simulink model "Manipulator"  (R2021a)
settings: Solver=VariableStepAuto  StartTime=0.0  StopTime=10.0  RelTol=1e-3
model workspace: external: MATLAB File /Users/nikodemlazarz/Documents/inzynierka/matlab/rotob /simscape/robot_DataFile.m (data not in the file)
undefined symbols (not defined in the file): S, smiData, Tx, Ty, Tz, X, x0, x1, Y, y0, y1, Z, z0, z1
libraries: sm_lib x20, simulink x8, nesl_utility x4
settings Model: Creator=nikod  LastModifiedBy=nikodemlazarz
settings ExplorerConfigSet: InternalSimMechanicsExplorerSettings="<ExplorerConfiguration><canonicalview>aerospace</canonicalview><AnimationSetting><BasePlaybackSpeed>1.0</BasePlaybackSpeed><PlaybackSpeedFactor>1.0</PlaybackSpeedFactor></AnimationSetting><TilePanel><TileInfo><Tiles Columns=\"1\" Count=\"1\" Rows=\"1\"><Column Weight=\"1\"/><Row Weight=\"1\"/><Tile Height=\"1\" Width=\"1\" X=\"0\" Y=\"0\"/></Tiles></TileInfo><SceneInfo><SceneViewer><BGColor><R>0.60000002384185791</R><G>0.60000002384185791</G><B>0.60000002384185791</B></BGColor><Camera><DoPerspective>off</DoPerspective><Position><X>2.62972255265206911</X><Y>-2.13592780536878957</Y><Z>-1.22972255243143036</Z></Position><Center><X>1.29999996897715486</X><Y>-0.806205221693875429</Y><Z>0.100000031243483445</Z></Center><Up><X>-0.408248290463863073</X><Y>0.408248290463863073</Y><Z>-0.816496580927726145</Z></Up><ViewLimDist>1</ViewLimDist><YLim>2.00898007835833559</YLim><XLim>1.8936319398880006</XLim></Camera></SceneViewer></SceneInfo></TilePanel><MechEditorPanel><Cameras/><GfxPanelCameraMap/><VideoCreator><PlaybackSpeedRatio>1.0</PlaybackSpeedRatio><FrameRate>30</FrameRate><VideoFormat>Motion JPEG AVI</VideoFormat><FrameSize>auto</FrameSize></VideoCreator></MechEditorPanel></ExplorerConfiguration>"

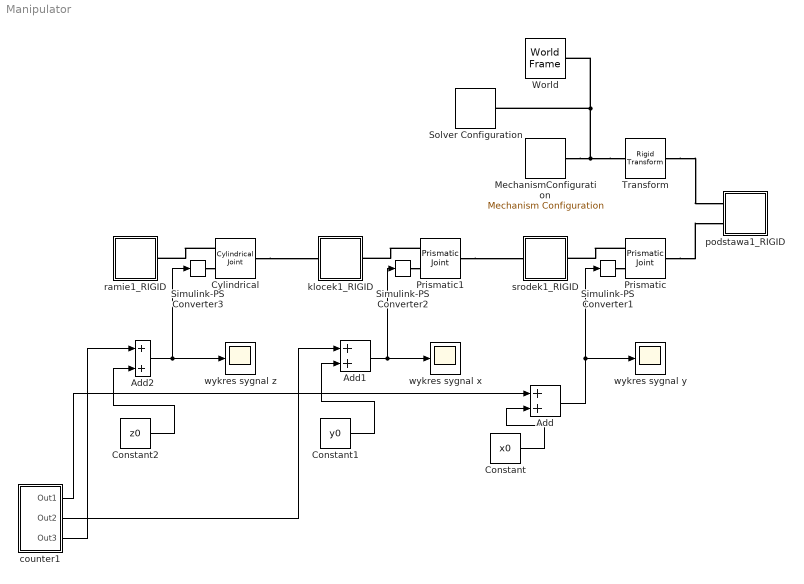
== system Manipulator ==
  Add : Sum
  Add1 : Sum
  Add2 : Sum
  Constant : Constant  Value=x0
  Constant1 : Constant  Value=y0
  Constant2 : Constant  Value=z0
  Cylindrical : sm_lib/Joints/Cylindrical Joint  JointMode=Normal  SenseConstraintForce=off  SenseConstraintForceX=off  SenseConstraintForceY=off  SenseConstraintForceZ=off  SenseConstraintTorque=off  SenseConstraintTorqueX=off  SenseConstraintTorqueY=off  SenseConstraintTorqueZ=off  SenseTotalForce=off  SenseTotalForceX=off  SenseTotalForceY=off  SenseTotalForceZ=off  SenseTotalTorque=off  SenseTotalTorqueX=off  SenseTotalTorqueY=off  SenseTotalTorqueZ=off  CompositeWrenchDir=FollowerOnBase  CompositeWrenchFrame=BaseFrame  PzEquilibriumPosition=0  PzEquilibriumPositionUnits=m  PzSpringStiffness=0  PzSpringStiffnessUnits=N/m  PzDampingCoefficient=0  PzDampingCoefficientUnits=N/(m/s)  PzTorqueActuationMode=ComputedTorque  PzMotionActuationMode=InputMotion  PzSensePosition=off  PzSenseVelocity=off  PzSenseAcceleration=off  PzSenseTorqueForce=off  PzSenseLowerLimitTorqueForce=off  PzSenseUpperLimitTorqueForce=off  PzLowerLimitSpecify=off  PzLowerLimitBound=-1  PzLowerLimitBoundUnits=m  PzLowerLimitStiffness=1e6  PzLowerLimitStiffnessUnits=N/m  PzLowerLimitDamping=1e3  PzLowerLimitDampingUnits=N/(m/s)  PzLowerLimitTransitionRegionWidth=1e-4  PzLowerLimitTransitionRegionWidthUnits=m  PzUpperLimitSpecify=off  PzUpperLimitBound=1  PzUpperLimitBoundUnits=m  PzUpperLimitStiffness=1e6  PzUpperLimitStiffnessUnits=N/m  PzUpperLimitDamping=1e3  PzUpperLimitDampingUnits=N/(m/s)  PzUpperLimitTransitionRegionWidth=1e-4  PzUpperLimitTransitionRegionWidthUnits=m  PzPositionTargetSpecify=on  PzPositionTargetPriority=Low  PzPositionTargetValue=z0  PzPositionTargetValueUnits=m  PzVelocityTargetSpecify=off  PzVelocityTargetPriority=High  PzVelocityTargetValue=0  PzVelocityTargetValueUnits=m/s  RzEquilibriumPosition=0  RzEquilibriumPositionUnits=deg  RzSpringStiffness=0  RzSpringStiffnessUnits=N*m/deg  RzDampingCoefficient=0  RzDampingCoefficientUnits=N*m/(deg/s)  RzTorqueActuationMode=NoTorque  RzMotionActuationMode=ComputedMotion  RzSensePosition=off  RzSenseVelocity=off  RzSenseAcceleration=off  RzSenseTorqueForce=off  RzSenseLowerLimitTorqueForce=off  RzSenseUpperLimitTorqueForce=off  RzLowerLimitSpecify=off  RzLowerLimitBound=-90  RzLowerLimitBoundUnits=deg  RzLowerLimitStiffness=1e4  RzLowerLimitStiffnessUnits=N*m/deg  RzLowerLimitDamping=10  RzLowerLimitDampingUnits=N*m/(deg/s)  RzLowerLimitTransitionRegionWidth=0.1  RzLowerLimitTransitionRegionWidthUnits=deg  RzUpperLimitSpecify=off  RzUpperLimitBound=90  RzUpperLimitBoundUnits=deg  RzUpperLimitStiffness=1e4  RzUpperLimitStiffnessUnits=N*m/deg  RzUpperLimitDamping=10  RzUpperLimitDampingUnits=N*m/(deg/s)  RzUpperLimitTransitionRegionWidth=0.1  RzUpperLimitTransitionRegionWidthUnits=deg  RzPositionTargetSpecify=on  RzPositionTargetPriority=Low  RzPositionTargetValue=smiData.CylindricalJoint(1).Rz.Pos  RzPositionTargetValueUnits=deg  RzVelocityTargetSpecify=off  RzVelocityTargetPriority=High  RzVelocityTargetValue=0  RzVelocityTargetValueUnits=deg/s
  MechanismConfiguration : sm_lib/Utilities/Mechanism Configuration  UniformGravity=Constant  GravityVector=[0 -9.80665 0]  GravityVectorUnits=m/s^2  GravityUnits=m/s^2  LinearizationDelta=0.001  JointModeTransitionNonlinearIterations=2
  Prismatic : sm_lib/Joints/Prismatic Joint  JointMode=Normal  SenseConstraintForce=off  SenseConstraintForceX=off  SenseConstraintForceY=off  SenseConstraintForceZ=off  SenseConstraintTorque=off  SenseConstraintTorqueX=off  SenseConstraintTorqueY=off  SenseConstraintTorqueZ=off  SenseTotalForce=off  SenseTotalForceX=off  SenseTotalForceY=off  SenseTotalForceZ=off  SenseTotalTorque=off  SenseTotalTorqueX=off  SenseTotalTorqueY=off  SenseTotalTorqueZ=off  CompositeWrenchDir=FollowerOnBase  CompositeWrenchFrame=BaseFrame  EquilibriumPosition=0  EquilibriumPositionUnits=m  SpringStiffness=0  SpringStiffnessUnits=N/m  DampingCoefficient=0  DampingCoefficientUnits=N/(m/s)  TorqueActuationMode=ComputedTorque  MotionActuationMode=InputMotion  SensePosition=off  SenseVelocity=off  SenseAcceleration=off  SenseTorqueForce=off  SenseLowerLimitTorqueForce=off  SenseUpperLimitTorqueForce=off  LowerLimitSpecify=off  LowerLimitBound=-1  LowerLimitBoundUnits=m  LowerLimitStiffness=1e6  LowerLimitStiffnessUnits=N/m  LowerLimitDamping=1e3  LowerLimitDampingUnits=N/(m/s)  LowerLimitTransitionRegionWidth=1e-4  LowerLimitTransitionRegionWidthUnits=m  UpperLimitSpecify=off  UpperLimitBound=1  UpperLimitBoundUnits=m  UpperLimitStiffness=1e6  UpperLimitStiffnessUnits=N/m  UpperLimitDamping=1e3  UpperLimitDampingUnits=N/(m/s)  UpperLimitTransitionRegionWidth=1e-4  UpperLimitTransitionRegionWidthUnits=m  PositionTargetSpecify=on  PositionTargetPriority=Low  PositionTargetValue=x0  PositionTargetValueUnits=m  VelocityTargetSpecify=off  VelocityTargetPriority=High  VelocityTargetValue=0  VelocityTargetValueUnits=m/s
  Prismatic1 : sm_lib/Joints/Prismatic Joint  JointMode=Normal  SenseConstraintForce=off  SenseConstraintForceX=off  SenseConstraintForceY=off  SenseConstraintForceZ=off  SenseConstraintTorque=off  SenseConstraintTorqueX=off  SenseConstraintTorqueY=off  SenseConstraintTorqueZ=off  SenseTotalForce=off  SenseTotalForceX=off  SenseTotalForceY=off  SenseTotalForceZ=off  SenseTotalTorque=off  SenseTotalTorqueX=off  SenseTotalTorqueY=off  SenseTotalTorqueZ=off  CompositeWrenchDir=FollowerOnBase  CompositeWrenchFrame=BaseFrame  EquilibriumPosition=0  EquilibriumPositionUnits=m  SpringStiffness=0  SpringStiffnessUnits=N/m  DampingCoefficient=0  DampingCoefficientUnits=N/(m/s)  TorqueActuationMode=ComputedTorque  MotionActuationMode=InputMotion  SensePosition=off  SenseVelocity=off  SenseAcceleration=off  SenseTorqueForce=off  SenseLowerLimitTorqueForce=off  SenseUpperLimitTorqueForce=off  LowerLimitSpecify=off  LowerLimitBound=-1  LowerLimitBoundUnits=m  LowerLimitStiffness=1e6  LowerLimitStiffnessUnits=N/m  LowerLimitDamping=1e3  LowerLimitDampingUnits=N/(m/s)  LowerLimitTransitionRegionWidth=1e-4  LowerLimitTransitionRegionWidthUnits=m  UpperLimitSpecify=off  UpperLimitBound=1  UpperLimitBoundUnits=m  UpperLimitStiffness=1e6  UpperLimitStiffnessUnits=N/m  UpperLimitDamping=1e3  UpperLimitDampingUnits=N/(m/s)  UpperLimitTransitionRegionWidth=1e-4  UpperLimitTransitionRegionWidthUnits=m  PositionTargetSpecify=on  PositionTargetPriority=Low  PositionTargetValue=y0  PositionTargetValueUnits=m  VelocityTargetSpecify=off  VelocityTargetPriority=High  VelocityTargetValue=0  VelocityTargetValueUnits=m/s
  Simulink-PS Converter1 : nesl_utility/Simulink-PS Converter  PhysicalDomain=network_engine_domain  SubClassName=ps_input  LeftPortType=input  RightPortType=output  PseudoPeriodic=off  Frequencies=[]  NoiseDistribution=none  NoiseParameters=[]  Unit=1  AffineConversion=off  FilteringAndDerivatives=zero  SimscapeFilterOrder=1  InputFilterTimeConstant=0.001  UdotUserProvided=0
      settings: SourceProductBaseCode=PW,SS
  Simulink-PS Converter2 : nesl_utility/Simulink-PS Converter  PhysicalDomain=network_engine_domain  SubClassName=ps_input  LeftPortType=input  RightPortType=output  PseudoPeriodic=off  Frequencies=[]  NoiseDistribution=none  NoiseParameters=[]  Unit=1  AffineConversion=off  FilteringAndDerivatives=zero  SimscapeFilterOrder=1  InputFilterTimeConstant=0.001  UdotUserProvided=0
      settings: SourceProductBaseCode=PW,SS
  Simulink-PS Converter3 : nesl_utility/Simulink-PS Converter  PhysicalDomain=network_engine_domain  SubClassName=ps_input  LeftPortType=input  RightPortType=output  PseudoPeriodic=off  Frequencies=[]  NoiseDistribution=none  NoiseParameters=[]  Unit=1  AffineConversion=off  FilteringAndDerivatives=zero  SimscapeFilterOrder=1  InputFilterTimeConstant=0.001  UdotUserProvided=0
      settings: SourceProductBaseCode=PW,SS
  Solver Configuration : nesl_utility/Solver Configuration  PhysicalDomain=network_engine_domain  SubClassName=solver  LeftPortType=input  RightPortType=generic  Tones=[]  Harmonics=[]  SimulateNoise=off  Profile=off  UseLocalSampling=off  EnableSwitchedLinearOptims=on  FrequencyDomain=off  UseCCode=off  RelTol=0.001  AbsTol=1e-06  MinStep=1e-09  ToWorkspace=off  RevertToSquareIcSolve=off  NumHomotopyIterations=100  PhasorMode=off  PhasorModeNumHarmonics=1  DoDC=off  ResidualTolerance=1e-09  UseLocalSolver=off  LocalSolverChoice=NE_BACKWARD_EULER_ADVANCER  LocalSolverSampleTime=0.001  DoFixedCost=off  MaxNonlinIter=3  MaxModeIter=2  ComputeImpulses=off  ImpulseIterations=2  LinearAlgebra=auto  EquationFormulation=NE_TIME_EF  DelaysMemoryBudget=1024  AutomaticFiltering=on  FilteringTimeConstant=0.001  PartitionStorageMethod=AS_NEEDED  PartitionMemoryBudget=1024  PartitionMethod=ROBUST
      settings: SourceProductBaseCode=PW,SS
  Transform : sm_lib/Frames and Transforms/Rigid Transform  TranslationMethod=Cartesian  TranslationStandardOffset=0  TranslationLengthUnit=mm  TranslationStandardAxis=+Z  TranslationCartesianOffset=smiData.RigidTransform(7).translation  TranslationROffset=0  TranslationROffsetUnits=m  TranslationZOffset=0  TranslationZOffsetUnits=m  TranslationThetaOffset=0  TranslationThetaOffsetUnits=deg  RotationMethod=ArbitraryAxis  RotationAngleUnits=rad  RotationStandardAxis=+Z  RotationAngle=smiData.RigidTransform(7).angle  RotationArbitraryAxis=smiData.RigidTransform(7).axis  FollAlignAxisA=+X  BaseAlignAxisA=+Y  FollAlignAxisB=+Y  BaseAlignAxisB=+Z  RotationSequenceAxes=FollowerAxes  RotationSequence=XYX  RotationSequenceAngles=[0 0 0]  RotationSequenceAnglesUnits=deg  RotationMatrix=[1 0 0; 0 1 0; 0 0 1]
  World : sm_lib/Frames and Transforms/World Frame
  counter1 : Subsystem
  klocek1_RIGID : Subsystem
  podstawa1_RIGID : Subsystem
  ramie1_RIGID : Subsystem
  srodek1_RIGID : Subsystem
  wykres sygnal x : Scope
  wykres sygnal y : Scope
  wykres sygnal z : Scope
  wires:
  Add1/1 -> wykres sygnal x/1, Simulink-PS Converter2/1
  Constant1/1 -> Add1/2
  Add2/1 -> Simulink-PS Converter3/1, wykres sygnal z/1
  Constant/1 -> Add/2
  Add/1 -> wykres sygnal y/1, Simulink-PS Converter1/1
  Constant2/1 -> Add2/2
  counter1/1(Out1) -> Add/1
  counter1/2(Out2) -> Add1/1
  counter1/3(Out3) -> Add2/1
  connections:
  Transform/LConn1 -- MechanismConfiguration/RConn1 -- World/RConn1 -- Solver Configuration/RConn1
  Prismatic/LConn1 -- srodek1_RIGID/RConn1
  Prismatic/RConn1 -- podstawa1_RIGID/LConn2
  Prismatic1/LConn1 -- klocek1_RIGID/RConn1
  Prismatic1/RConn1 -- srodek1_RIGID/LConn1
  Cylindrical/LConn1 -- ramie1_RIGID/RConn1
  Cylindrical/RConn1 -- klocek1_RIGID/LConn1
  Transform/RConn1 -- podstawa1_RIGID/LConn1
  Simulink-PS Converter1/RConn1 -- Prismatic/LConn2
  Simulink-PS Converter2/RConn1 -- Prismatic1/LConn2
  Simulink-PS Converter3/RConn1 -- Cylindrical/LConn2

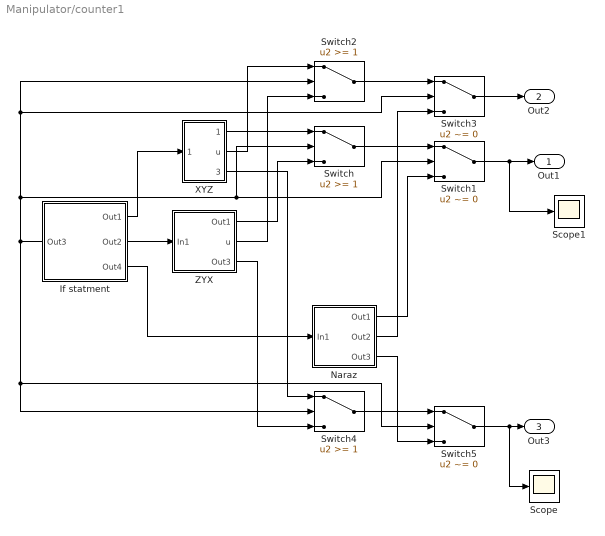
== system Manipulator/counter1 ==
  If statment : Subsystem
      settings: PortSchema="{\"entries\":[{\"content\":{\"sides\":[{\"content\":{\"connectorIds\":[\"Out4\"]},\"type\":\"ConnectorPlacement.EquallySpacedRectSide\",\"uuid\":\"055e23d9-8118-4299-bab5-0000c6d0c59b\"},{\"content\":{\"connectorIds\":[\"Out1\",\"Out2\",\"Out3\"],\"side\":\"RIGHT\"},\"type\":\"ConnectorPlacement.EquallySpacedRectSide\",\"uuid\":\"9d6ed615-8079-4081-ad2f-f5696b8bd135\"},{\"content\":{\"connectorIds\":[],\"side\":\"TOP\"},\"type\":\"ConnectorPlacement.EquallySpacedRectSide\",\"uuid\":\"f56795d6-4142-4a73-a6ec-9e1ccb17adc5\"}]},\"type\":\"ConnectorPlacement.EquallySpacedConnector\",\"uuid\":\"b4b5783c-fdb7-4a38-9420-ebfc82b5b324\"}],\"packageUris\":[\"http://schema.mathworks.com/mf0/Connector/R2020b\"],\"version\":\"1.0\"}"
  Naraz : Subsystem
  Scope : Scope
  Scope1 : Scope
  Switch : Switch  Threshold=1
  Switch1 : Switch  Criteria=u2 ~= 0
  Switch2 : Switch  Threshold=1
  Switch3 : Switch  Criteria=u2 ~= 0
  Switch4 : Switch  Threshold=1
  Switch5 : Switch  Criteria=u2 ~= 0
  XYZ : Subsystem
  ZYX : Subsystem
  Out1 : Outport
  Out2 : Outport  Port=2
  Out3 : Outport  Port=3
  wires:
  Naraz/2(Out2) -> Switch3/3
  Switch4/1 -> Switch5/1
  XYZ/2(u) -> Switch2/1
  If statment/2(Out2) -> ZYX/1(In1)
  Switch1/1 -> Scope1/1, Out1/1
  XYZ/1(Out1) -> Switch/1
  If statment/3(Out4) -> Naraz/1(In1)
  Switch3/1 -> Out2/1
  ZYX/2(u) -> Switch2/3
  Switch2/1 -> Switch3/1
  Switch/1 -> Switch1/1
  If statment/1(Out1) -> XYZ/1(In1)
  Switch5/1 -> Scope/1, Out3/1
  Naraz/3(Out3) -> Switch5/3
  ZYX/3(Out3) -> Switch4/3
  ZYX/1(Out1) -> Switch/3
  XYZ/3(Out3) -> Switch4/1
  Naraz/1(Out1) -> Switch1/3
  If statment/4(Out3) -> Switch5/2, Switch4/2, Switch1/2, Switch/2, Switch3/2, Switch2/2

== system Manipulator/klocek1_RIGID ==
  ReferenceFrame : sm_lib/Frames and Transforms/Reference Frame
  Transform : sm_lib/Frames and Transforms/Rigid Transform  TranslationMethod=Cartesian  TranslationStandardOffset=0  TranslationLengthUnit=mm  TranslationStandardAxis=+Z  TranslationCartesianOffset=smiData.RigidTransform(3).translation  TranslationROffset=0  TranslationROffsetUnits=m  TranslationZOffset=0  TranslationZOffsetUnits=m  TranslationThetaOffset=0  TranslationThetaOffsetUnits=deg  RotationMethod=ArbitraryAxis  RotationAngleUnits=rad  RotationStandardAxis=+Z  RotationAngle=smiData.RigidTransform(3).angle  RotationArbitraryAxis=smiData.RigidTransform(3).axis  FollAlignAxisA=+X  BaseAlignAxisA=+Y  FollAlignAxisB=+Y  BaseAlignAxisB=+Z  RotationSequenceAxes=FollowerAxes  RotationSequence=XYX  RotationSequenceAngles=[0 0 0]  RotationSequenceAnglesUnits=deg  RotationMatrix=[1 0 0; 0 1 0; 0 0 1]
  Transform1 : sm_lib/Frames and Transforms/Rigid Transform  TranslationMethod=Cartesian  TranslationStandardOffset=0  TranslationLengthUnit=mm  TranslationStandardAxis=+Z  TranslationCartesianOffset=smiData.RigidTransform(6).translation  TranslationROffset=0  TranslationROffsetUnits=m  TranslationZOffset=0  TranslationZOffsetUnits=m  TranslationThetaOffset=0  TranslationThetaOffsetUnits=deg  RotationMethod=ArbitraryAxis  RotationAngleUnits=rad  RotationStandardAxis=+Z  RotationAngle=smiData.RigidTransform(6).angle  RotationArbitraryAxis=smiData.RigidTransform(6).axis  FollAlignAxisA=+X  BaseAlignAxisA=+Y  FollAlignAxisB=+Y  BaseAlignAxisB=+Z  RotationSequenceAxes=FollowerAxes  RotationSequence=XYX  RotationSequenceAngles=[0 0 0]  RotationSequenceAnglesUnits=deg  RotationMatrix=[1 0 0; 0 1 0; 0 0 1]
  klocek : sm_lib/Body Elements/File Solid  ExtGeomFileName=/Users/nikodemlazarz/Documents/inzynierka/matlab/rotob /simscape/klocek_ipt_fa86c31d.STEP  UnitType=FromFile  ExtGeomFileUnits=m  StepReaderType=HEX  ExportConvexHullGeometry=off  InertiaType=Custom  Mass=smiData.Solid(3).mass  MassUnits=kg  CenterOfMass=smiData.Solid(3).CoM  CenterOfMassUnits=mm  MomentsOfInertia=smiData.Solid(3).MoI  MomentsOfInertiaUnits=kg*mm^2  ProductsOfInertia=smiData.Solid(3).PoI  ProductsOfInertiaUnits=kg*mm^2  BasedOnType=DensityFromFile  Density=1000  DensityUnits=kg/m^3  DoExposeReferenceFrame=on  SerializedFrames=<Frames/>  GraphicType=FromGeometry  MarkerShape=Sphere  MarkerSize=10  GraphicVisPropType=SimpleVisualProperties  GraphicDiffuseColor=smiData.Solid(3).color  GraphicSpecularColor=[0.5 0.5 0.5 1.0]  GraphicAmbientColor=[0.15 0.15 0.15 1.0]  GraphicEmissiveColor=[0.0 0.0 0.0 1.0]  GraphicShininess=75  GraphicOpacity=smiData.Solid(3).opacity
  F1 : PMIOPort  Side=Left
  F : PMIOPort  Port=2  Side=Right
  connections:
  klocek/RConn1 -- ReferenceFrame/RConn1 -- Transform/LConn1 -- Transform1/LConn1
  Transform/RConn1 -- F/RConn1
  Transform1/RConn1 -- F1/RConn1

== system Manipulator/podstawa1_RIGID ==
  Podstawa : sm_lib/Body Elements/File Solid  ExtGeomFileName=/Users/nikodemlazarz/Documents/inzynierka/matlab/rotob /simscape/podstawa_ipt_15195c3c.STEP  UnitType=FromFile  ExtGeomFileUnits=m  StepReaderType=HEX  ExportConvexHullGeometry=off  InertiaType=Custom  Mass=smiData.Solid(1).mass  MassUnits=kg  CenterOfMass=smiData.Solid(1).CoM  CenterOfMassUnits=mm  MomentsOfInertia=smiData.Solid(1).MoI  MomentsOfInertiaUnits=kg*mm^2  ProductsOfInertia=smiData.Solid(1).PoI  ProductsOfInertiaUnits=kg*mm^2  BasedOnType=DensityFromFile  Density=1000  DensityUnits=kg/m^3  DoExposeReferenceFrame=on  SerializedFrames=<Frames/>  GraphicType=FromGeometry  MarkerShape=Sphere  MarkerSize=10  GraphicVisPropType=SimpleVisualProperties  GraphicDiffuseColor=smiData.Solid(1).color  GraphicSpecularColor=[0.5 0.5 0.5 1.0]  GraphicAmbientColor=[0.15 0.15 0.15 1.0]  GraphicEmissiveColor=[0.0 0.0 0.0 1.0]  GraphicShininess=75  GraphicOpacity=smiData.Solid(1).opacity
  ReferenceFrame : sm_lib/Frames and Transforms/Reference Frame
  Transform : sm_lib/Frames and Transforms/Rigid Transform  TranslationMethod=Cartesian  TranslationStandardOffset=0  TranslationLengthUnit=mm  TranslationStandardAxis=+Z  TranslationCartesianOffset=smiData.RigidTransform(2).translation  TranslationROffset=0  TranslationROffsetUnits=m  TranslationZOffset=0  TranslationZOffsetUnits=m  TranslationThetaOffset=0  TranslationThetaOffsetUnits=deg  RotationMethod=ArbitraryAxis  RotationAngleUnits=rad  RotationStandardAxis=+Z  RotationAngle=smiData.RigidTransform(2).angle  RotationArbitraryAxis=smiData.RigidTransform(2).axis  FollAlignAxisA=+X  BaseAlignAxisA=+Y  FollAlignAxisB=+Y  BaseAlignAxisB=+Z  RotationSequenceAxes=FollowerAxes  RotationSequence=XYX  RotationSequenceAngles=[0 0 0]  RotationSequenceAnglesUnits=deg  RotationMatrix=[1 0 0; 0 1 0; 0 0 1]
  F1 : PMIOPort  Side=Left
  F : PMIOPort  Port=2  Side=Left
  connections:
  Podstawa/RConn1 -- ReferenceFrame/RConn1 -- Transform/LConn1 -- F1/RConn1
  Transform/RConn1 -- F/RConn1

== system Manipulator/ramie1_RIGID ==
  ReferenceFrame : sm_lib/Frames and Transforms/Reference Frame
  Transform : sm_lib/Frames and Transforms/Rigid Transform  TranslationMethod=Cartesian  TranslationStandardOffset=0  TranslationLengthUnit=mm  TranslationStandardAxis=+Z  TranslationCartesianOffset=smiData.RigidTransform(5).translation  TranslationROffset=0  TranslationROffsetUnits=m  TranslationZOffset=0  TranslationZOffsetUnits=m  TranslationThetaOffset=0  TranslationThetaOffsetUnits=deg  RotationMethod=ArbitraryAxis  RotationAngleUnits=rad  RotationStandardAxis=+Z  RotationAngle=smiData.RigidTransform(5).angle  RotationArbitraryAxis=smiData.RigidTransform(5).axis  FollAlignAxisA=+X  BaseAlignAxisA=+Y  FollAlignAxisB=+Y  BaseAlignAxisB=+Z  RotationSequenceAxes=FollowerAxes  RotationSequence=XYX  RotationSequenceAngles=[0 0 0]  RotationSequenceAnglesUnits=deg  RotationMatrix=[1 0 0; 0 1 0; 0 0 1]
  ramie : sm_lib/Body Elements/File Solid  ExtGeomFileName=/Users/nikodemlazarz/Documents/inzynierka/matlab/rotob /simscape/ramie_ipt_a44a51bd.STEP  UnitType=FromFile  ExtGeomFileUnits=m  StepReaderType=HEX  ExportConvexHullGeometry=off  InertiaType=Custom  Mass=smiData.Solid(4).mass  MassUnits=kg  CenterOfMass=smiData.Solid(4).CoM  CenterOfMassUnits=mm  MomentsOfInertia=smiData.Solid(4).MoI  MomentsOfInertiaUnits=kg*mm^2  ProductsOfInertia=smiData.Solid(4).PoI  ProductsOfInertiaUnits=kg*mm^2  BasedOnType=DensityFromFile  Density=1000  DensityUnits=kg/m^3  DoExposeReferenceFrame=on  SerializedFrames=<Frames/>  GraphicType=FromGeometry  MarkerShape=Sphere  MarkerSize=10  GraphicVisPropType=SimpleVisualProperties  GraphicDiffuseColor=smiData.Solid(4).color  GraphicSpecularColor=[0.5 0.5 0.5 1.0]  GraphicAmbientColor=[0.15 0.15 0.15 1.0]  GraphicEmissiveColor=[0.0 0.0 0.0 1.0]  GraphicShininess=75  GraphicOpacity=smiData.Solid(4).opacity
  F : PMIOPort  Side=Right
  connections:
  ramie/RConn1 -- ReferenceFrame/RConn1 -- Transform/LConn1
  Transform/RConn1 -- F/RConn1

== system Manipulator/srodek1_RIGID ==
  ReferenceFrame : sm_lib/Frames and Transforms/Reference Frame
  Transform : sm_lib/Frames and Transforms/Rigid Transform  TranslationMethod=Cartesian  TranslationStandardOffset=0  TranslationLengthUnit=mm  TranslationStandardAxis=+Z  TranslationCartesianOffset=smiData.RigidTransform(1).translation  TranslationROffset=0  TranslationROffsetUnits=m  TranslationZOffset=0  TranslationZOffsetUnits=m  TranslationThetaOffset=0  TranslationThetaOffsetUnits=deg  RotationMethod=ArbitraryAxis  RotationAngleUnits=rad  RotationStandardAxis=+Z  RotationAngle=smiData.RigidTransform(1).angle  RotationArbitraryAxis=smiData.RigidTransform(1).axis  FollAlignAxisA=+X  BaseAlignAxisA=+Y  FollAlignAxisB=+Y  BaseAlignAxisB=+Z  RotationSequenceAxes=FollowerAxes  RotationSequence=XYX  RotationSequenceAngles=[0 0 0]  RotationSequenceAnglesUnits=deg  RotationMatrix=[1 0 0; 0 1 0; 0 0 1]
  Transform1 : sm_lib/Frames and Transforms/Rigid Transform  TranslationMethod=Cartesian  TranslationStandardOffset=0  TranslationLengthUnit=mm  TranslationStandardAxis=+Z  TranslationCartesianOffset=smiData.RigidTransform(4).translation  TranslationROffset=0  TranslationROffsetUnits=m  TranslationZOffset=0  TranslationZOffsetUnits=m  TranslationThetaOffset=0  TranslationThetaOffsetUnits=deg  RotationMethod=ArbitraryAxis  RotationAngleUnits=rad  RotationStandardAxis=+Z  RotationAngle=smiData.RigidTransform(4).angle  RotationArbitraryAxis=smiData.RigidTransform(4).axis  FollAlignAxisA=+X  BaseAlignAxisA=+Y  FollAlignAxisB=+Y  BaseAlignAxisB=+Z  RotationSequenceAxes=FollowerAxes  RotationSequence=XYX  RotationSequenceAngles=[0 0 0]  RotationSequenceAnglesUnits=deg  RotationMatrix=[1 0 0; 0 1 0; 0 0 1]
  srodek : sm_lib/Body Elements/File Solid  ExtGeomFileName=/Users/nikodemlazarz/Documents/inzynierka/matlab/rotob /simscape/srodek_ipt_15195c3c.STEP  UnitType=FromFile  ExtGeomFileUnits=m  StepReaderType=HEX  ExportConvexHullGeometry=off  InertiaType=Custom  Mass=smiData.Solid(2).mass  MassUnits=kg  CenterOfMass=smiData.Solid(2).CoM  CenterOfMassUnits=mm  MomentsOfInertia=smiData.Solid(2).MoI  MomentsOfInertiaUnits=kg*mm^2  ProductsOfInertia=smiData.Solid(2).PoI  ProductsOfInertiaUnits=kg*mm^2  BasedOnType=DensityFromFile  Density=1000  DensityUnits=kg/m^3  DoExposeReferenceFrame=on  SerializedFrames=<Frames/>  GraphicType=FromGeometry  MarkerShape=Sphere  MarkerSize=10  GraphicVisPropType=SimpleVisualProperties  GraphicDiffuseColor=smiData.Solid(2).color  GraphicSpecularColor=[0.5 0.5 0.5 1.0]  GraphicAmbientColor=[0.15 0.15 0.15 1.0]  GraphicEmissiveColor=[0.0 0.0 0.0 1.0]  GraphicShininess=75  GraphicOpacity=smiData.Solid(2).opacity
  F1 : PMIOPort  Side=Left
  F : PMIOPort  Port=2  Side=Right
  connections:
  srodek/RConn1 -- ReferenceFrame/RConn1 -- Transform/LConn1 -- Transform1/LConn1
  Transform/RConn1 -- F/RConn1
  Transform1/RConn1 -- F1/RConn1

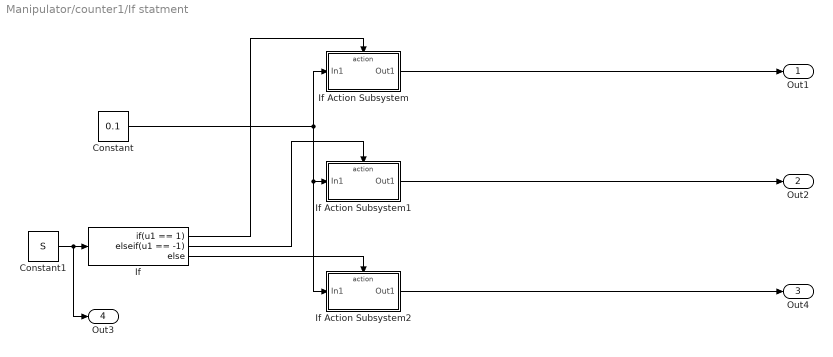
== system Manipulator/counter1/If statment ==
  Constant : Constant  Value=0.1
  Constant1 : Constant  Value=S
  If : If  IfExpression=u1 == 1  ElseIfExpressions=u1 == -1
  If Action Subsystem : Subsystem  TreatAsAtomicUnit=on
  If Action Subsystem1 : Subsystem  TreatAsAtomicUnit=on
  If Action Subsystem2 : Subsystem  TreatAsAtomicUnit=on
  Out1 : Outport
  Out2 : Outport  Port=2
  Out4 : Outport  Port=3
  Out3 : Outport  Port=4
  wires:
  Constant1/1 -> Out3/1, If/1
  If/3 -> If Action Subsystem2/Action
  Constant/1 -> If Action Subsystem/1(In1), If Action Subsystem2/1(In1), If Action Subsystem1/1(In1)
  If/2 -> If Action Subsystem1/Action
  If/1 -> If Action Subsystem/Action
  If Action Subsystem1/1(Out1) -> Out2/1
  If Action Subsystem/1(Out1) -> Out1/1
  If Action Subsystem2/1(Out1) -> Out4/1

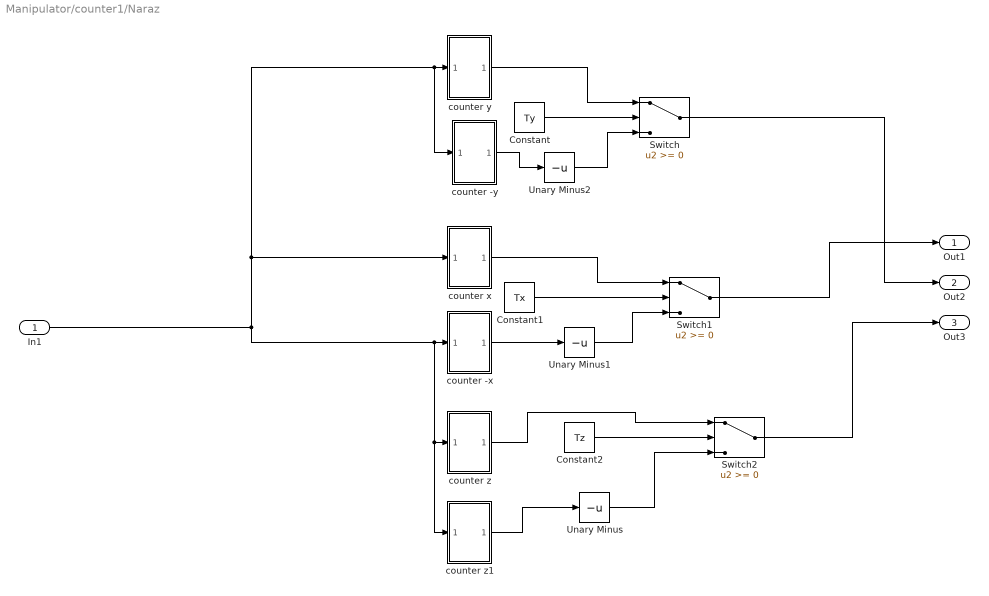
== system Manipulator/counter1/Naraz ==
  In1 : Inport
  Constant : Constant  Value=Ty
  Constant1 : Constant  Value=Tx
  Constant2 : Constant  Value=Tz
  Switch : Switch
  Switch1 : Switch
  Switch2 : Switch
  Unary Minus : UnaryMinus
  Unary Minus1 : UnaryMinus
  Unary Minus2 : UnaryMinus
  counter -x : Subsystem
  counter -y : Subsystem
  counter x : Subsystem
  counter y : Subsystem
  counter z : Subsystem
  counter z1 : Subsystem
  Out1 : Outport
  Out2 : Outport  Port=2
  Out3 : Outport  Port=3
  wires:
  Constant/1 -> Switch/2
  Unary Minus2/1 -> Switch/3
  Switch2/1 -> Out3/1
  counter z/1(Out3) -> Switch2/1
  counter -y/1(Out1) -> Unary Minus2/1
  counter -x/1(Out2) -> Unary Minus1/1
  Unary Minus1/1 -> Switch1/3
  Constant1/1 -> Switch1/2
  Unary Minus/1 -> Switch2/3
  counter x/1(Out2) -> Switch1/1
  In1/1 -> counter z1/1(In1), counter z/1(In1), counter -x/1(In1), counter x/1(In1), counter -y/1(In1), counter y/1(In1)
  Constant2/1 -> Switch2/2
  counter z1/1(Out3) -> Unary Minus/1
  counter y/1(Out1) -> Switch/1
  Switch1/1 -> Out1/1
  Switch/1 -> Out2/1

== system Manipulator/counter1/XYZ ==
  In1 : Inport
  Counter x : Subsystem
  Counter y : Subsystem
  Counter z : Subsystem
  "lacznik " : Subsystem
  lacznik x : Subsystem
  Out1 : Outport
  u : Outport  Port=2
  Out3 : Outport  Port=3
  wires:
  "lacznik "/1(Out1) -> Counter z/1(In1)
  Counter z/1(u) -> Out3/1
  lacznik x/1(u1) -> Counter y/1(u1), "lacznik "/2(u1)
  Counter x/1(u) -> Out1/1, lacznik x/1(u)
  In1/1 -> Counter x/1(In1)
  Counter y/1(u) -> u/1, "lacznik "/1(u)

== system Manipulator/counter1/ZYX ==
  In1 : Inport
  Counter x : Subsystem
  Counter y : Subsystem
  Counter z : Subsystem
  lacznik x : Subsystem
  lacznik z : Subsystem
  Out1 : Outport
  u : Outport  Port=2
  Out3 : Outport  Port=3
  wires:
  lacznik z/1(u1) -> Counter y/1(u1), lacznik x/2(u1)
  In1/1 -> Counter z/1(In1)
  Counter z/1(Out1) -> Out3/1, lacznik z/1(u)
  lacznik x/1(Out1) -> Counter x/1(In1)
  Counter x/1(Out1) -> Out1/1
  Counter y/1(u) -> u/1, lacznik x/1(u)

== system Manipulator/counter1/If statment/If Action Subsystem ==
  In1 : Inport
  Action Port : ActionPort  ActionPortLabel=if(u1 == 1)
  Out1 : Outport
  wires:
  In1/1 -> Out1/1

== system Manipulator/counter1/If statment/If Action Subsystem1 ==
  In1 : Inport
  Action Port : ActionPort  ActionPortLabel=elseif(u1 == -1)
  Out1 : Outport
  wires:
  In1/1 -> Out1/1

== system Manipulator/counter1/If statment/If Action Subsystem2 ==
  In1 : Inport
  Action Port : ActionPort  ActionPortLabel=else
  Out1 : Outport
  wires:
  In1/1 -> Out1/1

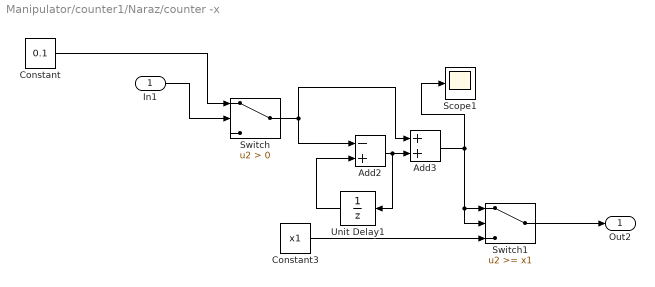
== system Manipulator/counter1/Naraz/counter -x ==
  In1 : Inport
  Add2 : Sum  Inputs=-+
  Add3 : Sum
  Constant : Constant  Value=0.1
  Constant3 : Constant  Value=x1
  Scope1 : Scope
  Switch : Switch  Criteria=u2 > Threshold
  Switch1 : Switch  Threshold=x1
  Unit Delay1 : UnitDelay  SampleTime=0.1  HasFrameUpgradeWarning=on
  Out2 : Outport
  wires:
  Add2/1 -> Unit Delay1/1, Add3/2
  Switch/1 -> Add3/1, Add2/1
  Switch1/1 -> Out2/1
  Add3/1 -> Switch1/2, Switch1/1, Scope1/1
  Constant3/1 -> Switch1/3
  Unit Delay1/1 -> Add2/2
  In1/1 -> Switch/2
  Constant/1 -> Switch/1

== system Manipulator/counter1/Naraz/counter -y ==
  In1 : Inport
  Add : Sum  Inputs=-+
  Add1 : Sum
  Constant1 : Constant  Value=y1
  Scope : Scope
  Switch : Switch  Threshold=y1
  Unit Delay : UnitDelay  SampleTime=0.1  HasFrameUpgradeWarning=on
  Out1 : Outport
  wires:
  Switch/1 -> Out1/1
  Unit Delay/1 -> Add/2
  Add/1 -> Unit Delay/1, Add1/2
  Add1/1 -> Scope/1, Switch/2, Switch/1
  Constant1/1 -> Switch/3
  In1/1 -> Add/1, Add1/1

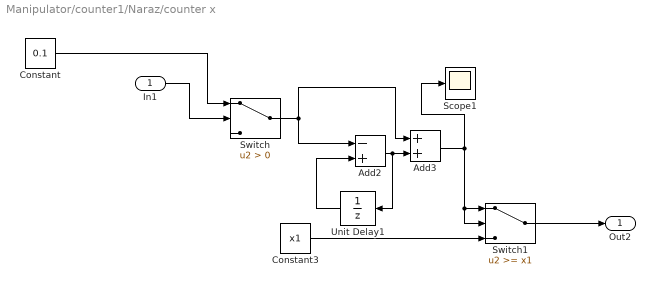
== system Manipulator/counter1/Naraz/counter x ==
  In1 : Inport
  Add2 : Sum  Inputs=-+
  Add3 : Sum
  Constant : Constant  Value=0.1
  Constant3 : Constant  Value=x1
  Scope1 : Scope
  Switch : Switch  Criteria=u2 > Threshold
  Switch1 : Switch  Threshold=x1
  Unit Delay1 : UnitDelay  SampleTime=0.1  HasFrameUpgradeWarning=on
  Out2 : Outport
  wires:
  Add2/1 -> Unit Delay1/1, Add3/2
  Switch/1 -> Add3/1, Add2/1
  Switch1/1 -> Out2/1
  Add3/1 -> Switch1/2, Switch1/1, Scope1/1
  Constant3/1 -> Switch1/3
  Unit Delay1/1 -> Add2/2
  In1/1 -> Switch/2
  Constant/1 -> Switch/1

== system Manipulator/counter1/Naraz/counter y ==
  In1 : Inport
  Add : Sum  Inputs=-+
  Add1 : Sum
  Constant1 : Constant  Value=y1
  Scope : Scope
  Switch : Switch  Threshold=y1
  Unit Delay : UnitDelay  SampleTime=0.1  HasFrameUpgradeWarning=on
  Out1 : Outport
  wires:
  Switch/1 -> Out1/1
  Unit Delay/1 -> Add/2
  Add/1 -> Unit Delay/1, Add1/2
  Add1/1 -> Scope/1, Switch/2, Switch/1
  Constant1/1 -> Switch/3
  In1/1 -> Add/1, Add1/1

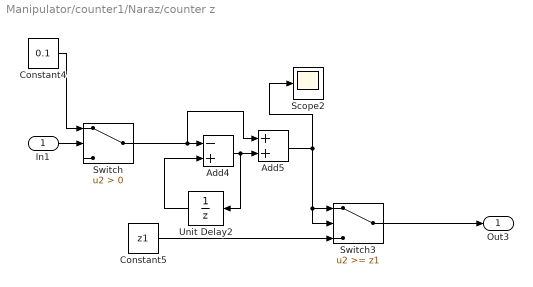
== system Manipulator/counter1/Naraz/counter z ==
  In1 : Inport
  Add4 : Sum  Inputs=-+
  Add5 : Sum
  Constant4 : Constant  Value=0.1
  Constant5 : Constant  Value=z1
  Scope2 : Scope
  Switch : Switch  Criteria=u2 > Threshold
  Switch3 : Switch  Threshold=z1
  Unit Delay2 : UnitDelay  SampleTime=0.1  HasFrameUpgradeWarning=on
  Out3 : Outport
  wires:
  Add5/1 -> Switch3/2, Switch3/1, Scope2/1
  Add4/1 -> Unit Delay2/1, Add5/2
  Constant5/1 -> Switch3/3
  Switch3/1 -> Out3/1
  Unit Delay2/1 -> Add4/2
  Constant4/1 -> Switch/1
  Switch/1 -> Add5/1, Add4/1
  In1/1 -> Switch/2

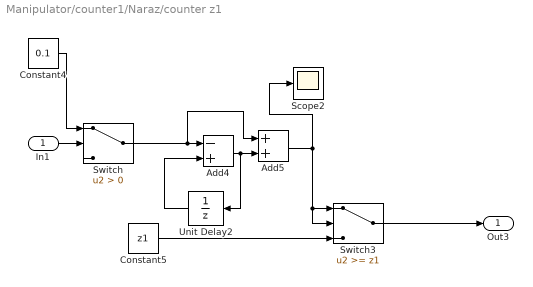
== system Manipulator/counter1/Naraz/counter z1 ==
  In1 : Inport
  Add4 : Sum  Inputs=-+
  Add5 : Sum
  Constant4 : Constant  Value=0.1
  Constant5 : Constant  Value=z1
  Scope2 : Scope
  Switch : Switch  Criteria=u2 > Threshold
  Switch3 : Switch  Threshold=z1
  Unit Delay2 : UnitDelay  SampleTime=0.1  HasFrameUpgradeWarning=on
  Out3 : Outport
  wires:
  Add5/1 -> Switch3/2, Switch3/1, Scope2/1
  Add4/1 -> Unit Delay2/1, Add5/2
  Constant5/1 -> Switch3/3
  Switch3/1 -> Out3/1
  Unit Delay2/1 -> Add4/2
  Constant4/1 -> Switch/1
  Switch/1 -> Add5/1, Add4/1
  In1/1 -> Switch/2

== system Manipulator/counter1/XYZ/Counter x ==
  In1 : Inport
  Constant1 : Constant  Value=Tx
  Scope : Scope
  Switch1 : Switch
  Unary Minus1 : UnaryMinus
  counter -x : Subsystem
  counter x : Subsystem
  u : Outport
  wires:
  In1/1 -> counter x/1(In1), counter -x/1(In1)
  counter -x/1(Out2) -> Unary Minus1/1
  Constant1/1 -> Switch1/2
  Switch1/1 -> Scope/1, u/1
  Unary Minus1/1 -> Switch1/3
  counter x/1(Out2) -> Switch1/1

== system Manipulator/counter1/XYZ/Counter y ==
  u1 : Inport
  Constant1 : Constant  Value=Ty
  Scope : Scope
  Switch1 : Switch
  Unary Minus1 : UnaryMinus
  counter -y : Subsystem
  counter y : Subsystem
  u : Outport
  wires:
  u1/1 -> counter y/1(In1), counter -y/1(In1)
  counter -y/1(Out2) -> Unary Minus1/1
  Constant1/1 -> Switch1/2
  Switch1/1 -> u/1
  Unary Minus1/1 -> Scope/1, Switch1/3
  counter y/1(Out2) -> Switch1/1

== system Manipulator/counter1/XYZ/Counter z ==
  In1 : Inport
  Constant1 : Constant  Value=Tz
  Switch1 : Switch
  Unary Minus1 : UnaryMinus
  counter -z : Subsystem
  counter z : Subsystem
  u : Outport
  wires:
  In1/1 -> counter z/1(In1), counter -z/1(In1)
  counter -z/1(Out2) -> Unary Minus1/1
  Constant1/1 -> Switch1/2
  Switch1/1 -> u/1
  Unary Minus1/1 -> Switch1/3
  counter z/1(Out2) -> Switch1/1

== system Manipulator/counter1/XYZ/lacznik  ==
  u : Inport
  u1 : Inport  Port=2
  Add : Sum
  Compare To Constant : simulink/Logic and Bit Operations/Compare To Constant  relop===  const=y1  OutDataTypeStr=boolean
  Compare To Constant1 : simulink/Logic and Bit Operations/Compare To Constant  relop===  const=-y1  OutDataTypeStr=boolean
  Logical Operator : Logic  AllPortsSameDT=off  OutDataTypeStr=boolean
  Out1 : Outport
  wires:
  Compare To Constant1/1 -> Add/2
  u/1 -> Compare To Constant/1, Compare To Constant1/1
  Compare To Constant/1 -> Add/1
  u1/1 -> Logical Operator/2
  Add/1 -> Logical Operator/1
  Logical Operator/1 -> Out1/1

== system Manipulator/counter1/XYZ/lacznik x ==
  u : Inport
  Add : Sum
  Compare To Constant : simulink/Logic and Bit Operations/Compare To Constant  relop===  const=x1  OutDataTypeStr=boolean
  Compare To Constant1 : simulink/Logic and Bit Operations/Compare To Constant  relop===  const=-x1  OutDataTypeStr=boolean
  u1 : Outport
  wires:
  Compare To Constant1/1 -> Add/2
  u/1 -> Compare To Constant/1, Compare To Constant1/1
  Compare To Constant/1 -> Add/1
  Add/1 -> u1/1

== system Manipulator/counter1/ZYX/Counter x ==
  In1 : Inport
  Constant1 : Constant  Value=Tx
  Switch1 : Switch
  Unary Minus1 : UnaryMinus
  counter -x : Subsystem
  counter x : Subsystem
  Out1 : Outport
  wires:
  In1/1 -> counter x/1(In1), counter -x/1(In1)
  counter -x/1(Out2) -> Unary Minus1/1
  Constant1/1 -> Switch1/2
  Switch1/1 -> Out1/1
  Unary Minus1/1 -> Switch1/3
  counter x/1(Out2) -> Switch1/1

== system Manipulator/counter1/ZYX/Counter y ==
  u1 : Inport
  Constant1 : Constant  Value=Ty
  Switch1 : Switch
  Unary Minus1 : UnaryMinus
  counter -y : Subsystem
  counter y : Subsystem
  u : Outport
  wires:
  u1/1 -> counter y/1(In1), counter -y/1(In1)
  counter -y/1(Out2) -> Unary Minus1/1
  Constant1/1 -> Switch1/2
  Switch1/1 -> u/1
  Unary Minus1/1 -> Switch1/3
  counter y/1(Out2) -> Switch1/1

== system Manipulator/counter1/ZYX/Counter z ==
  In1 : Inport
  Constant2 : Constant  Value=Tz
  Switch2 : Switch
  Unary Minus : UnaryMinus
  counter -z : Subsystem
  counter z : Subsystem
  Out1 : Outport
  wires:
  Constant2/1 -> Switch2/2
  In1/1 -> counter -z/1(In1), counter z/1(In1)
  Switch2/1 -> Out1/1
  counter z/1(Out3) -> Switch2/1
  Unary Minus/1 -> Switch2/3
  counter -z/1(Out3) -> Unary Minus/1

== system Manipulator/counter1/ZYX/lacznik x ==
  u : Inport
  u1 : Inport  Port=2
  AND : Logic  AllPortsSameDT=off  OutDataTypeStr=boolean
  Add : Sum
  Compare To Constant : simulink/Logic and Bit Operations/Compare To Constant  relop===  const=y1  OutDataTypeStr=boolean
  Compare To Constant1 : simulink/Logic and Bit Operations/Compare To Constant  relop===  const=-y1  OutDataTypeStr=boolean
  Out1 : Outport
  wires:
  Compare To Constant1/1 -> Add/2
  u/1 -> Compare To Constant/1, Compare To Constant1/1
  Compare To Constant/1 -> Add/1
  AND/1 -> Out1/1
  Add/1 -> AND/1
  u1/1 -> AND/2

== system Manipulator/counter1/ZYX/lacznik z ==
  u : Inport
  Add : Sum
  Compare To Constant : simulink/Logic and Bit Operations/Compare To Constant  relop===  const=z1  OutDataTypeStr=boolean
  Compare To Constant1 : simulink/Logic and Bit Operations/Compare To Constant  relop===  const=-z1  OutDataTypeStr=boolean
  u1 : Outport
  wires:
  Compare To Constant1/1 -> Add/2
  u/1 -> Compare To Constant/1, Compare To Constant1/1
  Compare To Constant/1 -> Add/1
  Add/1 -> u1/1

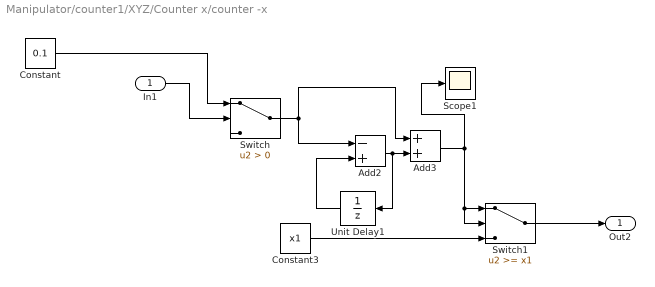
== system Manipulator/counter1/XYZ/Counter x/counter -x ==
  In1 : Inport
  Add2 : Sum  Inputs=-+
  Add3 : Sum
  Constant : Constant  Value=0.1
  Constant3 : Constant  Value=x1
  Scope1 : Scope
  Switch : Switch  Criteria=u2 > Threshold
  Switch1 : Switch  Threshold=x1
  Unit Delay1 : UnitDelay  SampleTime=0.1  HasFrameUpgradeWarning=on
  Out2 : Outport
  wires:
  Add2/1 -> Unit Delay1/1, Add3/2
  Switch/1 -> Add3/1, Add2/1
  Switch1/1 -> Out2/1
  Add3/1 -> Switch1/2, Switch1/1, Scope1/1
  Constant3/1 -> Switch1/3
  Unit Delay1/1 -> Add2/2
  In1/1 -> Switch/2
  Constant/1 -> Switch/1

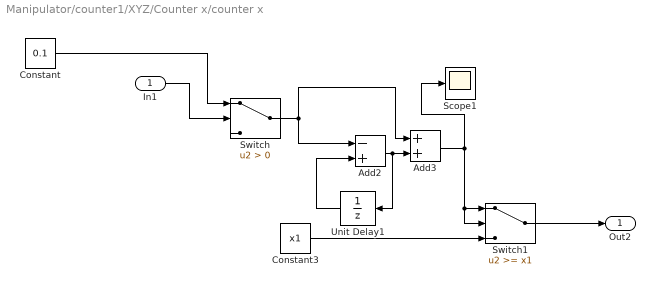
== system Manipulator/counter1/XYZ/Counter x/counter x ==
  In1 : Inport
  Add2 : Sum  Inputs=-+
  Add3 : Sum
  Constant : Constant  Value=0.1
  Constant3 : Constant  Value=x1
  Scope1 : Scope
  Switch : Switch  Criteria=u2 > Threshold
  Switch1 : Switch  Threshold=x1
  Unit Delay1 : UnitDelay  SampleTime=0.1  HasFrameUpgradeWarning=on
  Out2 : Outport
  wires:
  Add2/1 -> Unit Delay1/1, Add3/2
  Switch/1 -> Add3/1, Add2/1
  Switch1/1 -> Out2/1
  Add3/1 -> Switch1/2, Switch1/1, Scope1/1
  Constant3/1 -> Switch1/3
  Unit Delay1/1 -> Add2/2
  In1/1 -> Switch/2
  Constant/1 -> Switch/1

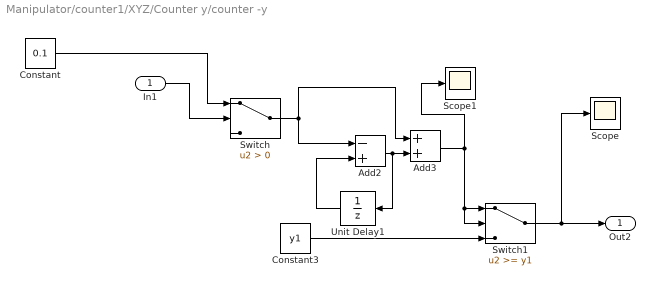
== system Manipulator/counter1/XYZ/Counter y/counter -y ==
  In1 : Inport
  Add2 : Sum  Inputs=-+
  Add3 : Sum
  Constant : Constant  Value=0.1
  Constant3 : Constant  Value=y1
  Scope : Scope
  Scope1 : Scope
  Switch : Switch  Criteria=u2 > Threshold
  Switch1 : Switch  Threshold=y1
  Unit Delay1 : UnitDelay  SampleTime=0.1  HasFrameUpgradeWarning=on
  Out2 : Outport
  wires:
  Add2/1 -> Unit Delay1/1, Add3/2
  Switch/1 -> Add3/1, Add2/1
  Switch1/1 -> Scope/1, Out2/1
  Add3/1 -> Switch1/2, Switch1/1, Scope1/1
  Constant3/1 -> Switch1/3
  Unit Delay1/1 -> Add2/2
  In1/1 -> Switch/2
  Constant/1 -> Switch/1

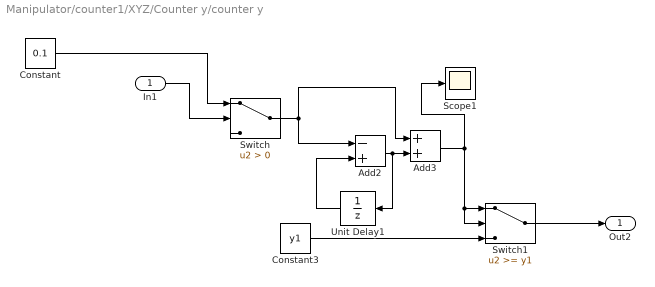
== system Manipulator/counter1/XYZ/Counter y/counter y ==
  In1 : Inport
  Add2 : Sum  Inputs=-+
  Add3 : Sum
  Constant : Constant  Value=0.1
  Constant3 : Constant  Value=y1
  Scope1 : Scope
  Switch : Switch  Criteria=u2 > Threshold
  Switch1 : Switch  Threshold=y1
  Unit Delay1 : UnitDelay  SampleTime=0.1  HasFrameUpgradeWarning=on
  Out2 : Outport
  wires:
  Add2/1 -> Unit Delay1/1, Add3/2
  Switch/1 -> Add3/1, Add2/1
  Switch1/1 -> Out2/1
  Add3/1 -> Switch1/2, Switch1/1, Scope1/1
  Constant3/1 -> Switch1/3
  Unit Delay1/1 -> Add2/2
  In1/1 -> Switch/2
  Constant/1 -> Switch/1

== system Manipulator/counter1/XYZ/Counter z/counter -z ==
  In1 : Inport
  Add2 : Sum  Inputs=-+
  Add3 : Sum
  Constant : Constant  Value=0.1
  Constant3 : Constant  Value=z1
  Scope1 : Scope
  Switch : Switch  Criteria=u2 > Threshold
  Switch1 : Switch  Threshold=z1
  Unit Delay1 : UnitDelay  SampleTime=0.1  HasFrameUpgradeWarning=on
  Out2 : Outport
  wires:
  Add2/1 -> Unit Delay1/1, Add3/2
  Switch/1 -> Add3/1, Add2/1
  Switch1/1 -> Out2/1
  Add3/1 -> Switch1/2, Switch1/1, Scope1/1
  Constant3/1 -> Switch1/3
  Unit Delay1/1 -> Add2/2
  In1/1 -> Switch/2
  Constant/1 -> Switch/1

== system Manipulator/counter1/XYZ/Counter z/counter z ==
  In1 : Inport
  Add2 : Sum  Inputs=-+
  Add3 : Sum
  Constant : Constant  Value=0.1
  Constant3 : Constant  Value=z1
  Scope1 : Scope
  Switch : Switch  Criteria=u2 > Threshold
  Switch1 : Switch  Threshold=z1
  Unit Delay1 : UnitDelay  SampleTime=0.1  HasFrameUpgradeWarning=on
  Out2 : Outport
  wires:
  Add2/1 -> Unit Delay1/1, Add3/2
  Switch/1 -> Add3/1, Add2/1
  Switch1/1 -> Out2/1
  Add3/1 -> Switch1/2, Switch1/1, Scope1/1
  Constant3/1 -> Switch1/3
  Unit Delay1/1 -> Add2/2
  In1/1 -> Switch/2
  Constant/1 -> Switch/1

== system Manipulator/counter1/ZYX/Counter x/counter -x ==
  In1 : Inport
  Add2 : Sum  Inputs=-+
  Add3 : Sum
  Constant : Constant  Value=0.1
  Constant3 : Constant  Value=x1
  Scope1 : Scope
  Switch : Switch  Criteria=u2 > Threshold
  Switch1 : Switch  Threshold=x1
  Unit Delay1 : UnitDelay  SampleTime=0.1  HasFrameUpgradeWarning=on
  Out2 : Outport
  wires:
  Add2/1 -> Unit Delay1/1, Add3/2
  Switch/1 -> Add3/1, Add2/1
  Switch1/1 -> Out2/1
  Add3/1 -> Switch1/2, Switch1/1, Scope1/1
  Constant3/1 -> Switch1/3
  Unit Delay1/1 -> Add2/2
  In1/1 -> Switch/2
  Constant/1 -> Switch/1

== system Manipulator/counter1/ZYX/Counter x/counter x ==
  In1 : Inport
  Add2 : Sum  Inputs=-+
  Add3 : Sum
  Constant : Constant  Value=0.1
  Constant3 : Constant  Value=x1
  Scope1 : Scope
  Switch : Switch  Criteria=u2 > Threshold
  Switch1 : Switch  Threshold=x1
  Unit Delay1 : UnitDelay  SampleTime=0.1  HasFrameUpgradeWarning=on
  Out2 : Outport
  wires:
  Add2/1 -> Unit Delay1/1, Add3/2
  Switch/1 -> Add3/1, Add2/1
  Switch1/1 -> Out2/1
  Add3/1 -> Switch1/2, Switch1/1, Scope1/1
  Constant3/1 -> Switch1/3
  Unit Delay1/1 -> Add2/2
  In1/1 -> Switch/2
  Constant/1 -> Switch/1

== system Manipulator/counter1/ZYX/Counter y/counter -y ==
  In1 : Inport
  Add2 : Sum  Inputs=-+
  Add3 : Sum
  Constant : Constant  Value=0.1
  Constant3 : Constant  Value=y1
  Scope1 : Scope
  Switch : Switch  Criteria=u2 > Threshold
  Switch1 : Switch  Threshold=y1
  Unit Delay1 : UnitDelay  SampleTime=0.1  HasFrameUpgradeWarning=on
  Out2 : Outport
  wires:
  Add2/1 -> Unit Delay1/1, Add3/2
  Switch/1 -> Add3/1, Add2/1
  Switch1/1 -> Out2/1
  Add3/1 -> Switch1/2, Switch1/1, Scope1/1
  Constant3/1 -> Switch1/3
  Unit Delay1/1 -> Add2/2
  In1/1 -> Switch/2
  Constant/1 -> Switch/1

== system Manipulator/counter1/ZYX/Counter y/counter y ==
  In1 : Inport
  Add2 : Sum  Inputs=-+
  Add3 : Sum
  Constant : Constant  Value=0.1
  Constant3 : Constant  Value=y1
  Scope1 : Scope
  Switch : Switch  Criteria=u2 > Threshold
  Switch1 : Switch  Threshold=y1
  Unit Delay1 : UnitDelay  SampleTime=0.1  HasFrameUpgradeWarning=on
  Out2 : Outport
  wires:
  Add2/1 -> Unit Delay1/1, Add3/2
  Switch/1 -> Add3/1, Add2/1
  Switch1/1 -> Out2/1
  Add3/1 -> Switch1/2, Switch1/1, Scope1/1
  Constant3/1 -> Switch1/3
  Unit Delay1/1 -> Add2/2
  In1/1 -> Switch/2
  Constant/1 -> Switch/1

== system Manipulator/counter1/ZYX/Counter z/counter -z ==
  In1 : Inport
  Add4 : Sum  Inputs=-+
  Add5 : Sum
  Constant4 : Constant  Value=0.1
  Constant5 : Constant  Value=z1
  Scope2 : Scope
  Switch : Switch  Criteria=u2 > Threshold
  Switch3 : Switch  Threshold=z1
  Unit Delay2 : UnitDelay  SampleTime=0.1  HasFrameUpgradeWarning=on
  Out3 : Outport
  wires:
  Add5/1 -> Switch3/2, Switch3/1, Scope2/1
  Add4/1 -> Unit Delay2/1, Add5/2
  Constant5/1 -> Switch3/3
  Switch3/1 -> Out3/1
  Unit Delay2/1 -> Add4/2
  Constant4/1 -> Switch/1
  Switch/1 -> Add5/1, Add4/1
  In1/1 -> Switch/2

== system Manipulator/counter1/ZYX/Counter z/counter z ==
  In1 : Inport
  Add4 : Sum  Inputs=-+
  Add5 : Sum
  Constant4 : Constant  Value=0.1
  Constant5 : Constant  Value=z1
  Scope2 : Scope
  Switch : Switch  Criteria=u2 > Threshold
  Switch3 : Switch  Threshold=z1
  Unit Delay2 : UnitDelay  SampleTime=0.1  HasFrameUpgradeWarning=on
  Out3 : Outport
  wires:
  Add5/1 -> Switch3/2, Switch3/1, Scope2/1
  Add4/1 -> Unit Delay2/1, Add5/2
  Constant5/1 -> Switch3/3
  Switch3/1 -> Out3/1
  Unit Delay2/1 -> Add4/2
  Constant4/1 -> Switch/1
  Switch/1 -> Add5/1, Add4/1
  In1/1 -> Switch/2
